simulink subsystem "tehrani_rs_calculations"  (R2020b)
settings: Solver=VariableStepAuto  StartTime=0.0  StopTime=10.0  RelTol=1e-3
values from neighbouring files (symbols this model uses):
  C_a_CO2_0 = 0.54    [model_workspace.mat]
  C_a_O2_0 = 0.1974    [model_workspace.mat]
  C_v_CO2_0 = 0.72    [model_workspace.mat]
  C_v_O2_0 = 0.13    [model_workspace.mat]
  delay_arterial = 10    [model_workspace.mat]
  delay_venous = 0    [model_workspace.mat]
settings Model: Creator=RH  LastModifiedBy=fonck

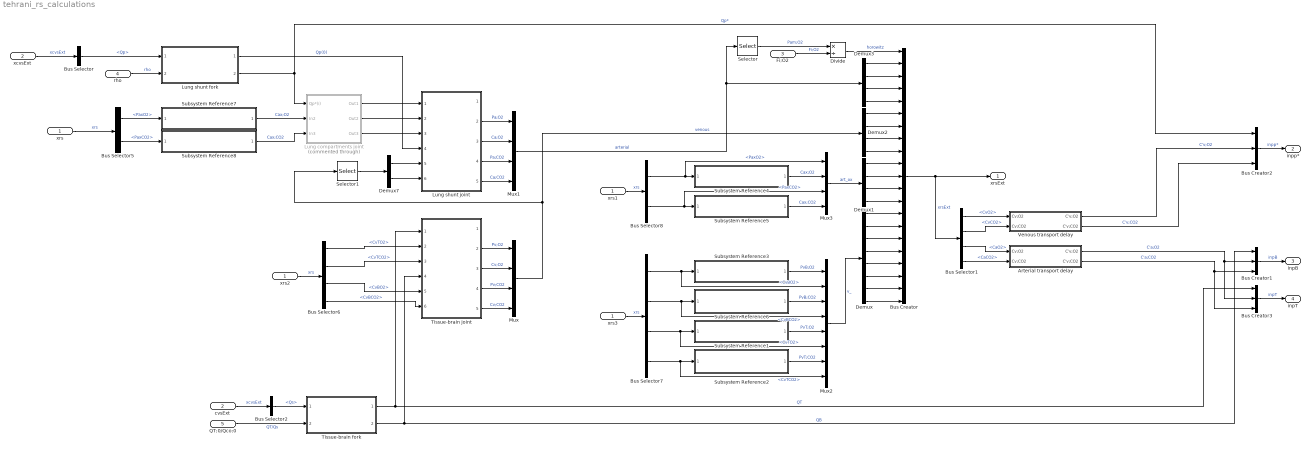
== system tehrani_rs_calculations ==
  xrs3 : Inport  OutDataTypeStr=Bus: RespiratoryState  Unit=liter/minute
  xcvsExt : Inport  Port=2  OutDataTypeStr=Bus: CardioVascularStateExtended  Unit=liter/minute
  Fi;O2 : Inport  Port=3  Unit=1
  rho : Inport  Port=4  Unit=1
  QT;0/Qco;0 : Inport  Port=5  Unit=1
  Arterial transport delay : Subsystem
  Bus Creator : BusCreator  Inputs=21  OutDataTypeStr=Bus: RespiratoryStateExtended
      settings: InheritFromInputs=off
  Bus Creator1 : BusCreator  Inputs=3  OutDataTypeStr=Bus: BloodGasFlow
      settings: InheritFromInputs=off
  Bus Creator2 : BusCreator  Inputs=3  OutDataTypeStr=Bus: BloodGasFlow
      settings: InheritFromInputs=off
  Bus Creator3 : BusCreator  Inputs=3  OutDataTypeStr=Bus: BloodGasFlow
      settings: InheritFromInputs=off
  Bus Selector : BusSelector  OutputSignals=Qp
  Bus Selector1 : BusSelector  OutputSignals=CvO2,CvCO2,CaO2,CaCO2
  Bus Selector2 : BusSelector  OutputSignals=Qs
  Bus Selector5 : BusSelector  OutputSignals=PaxO2,PaxCO2
  Bus Selector6 : BusSelector  OutputSignals=CvTO2,CvTCO2,CvBO2,CvBCO2
  Bus Selector7 : BusSelector  OutputSignals=CvBO2,CvBCO2,CvTO2,CvTCO2
  Bus Selector8 : BusSelector  OutputSignals=PaxO2,PaxCO2
  Demux : Demux  Outputs=8
  Demux1 : Demux
  Demux2 : Demux
  Demux3 : Demux
  Demux7 : Demux  Outputs=2
  Divide : Product  Inputs=*/
  Lung compartments joint : Subsystem  Commented=through
  Lung shunt fork : Subsystem  ReferencedSubsystem=blood_fork
  Lung shunt joint : Subsystem  ReferencedSubsystem=blood_joint
  Mux : Mux
  Mux1 : Mux
  Mux2 : Mux  Inputs=8
  Mux3 : Mux
  Selector : Selector  InputPortWidth=4  IndexOptions=Index vector (dialog)  Indices=[1]  OutputSizes=1
  Selector1 : Selector  InputPortWidth=4  IndexOptions=Index vector (dialog)  Indices=[2 4]  OutputSizes=1
  Subsystem Reference1 : Subsystem  ReferencedSubsystem=O2_dissociation_inv
  Subsystem Reference2 : Subsystem  ReferencedSubsystem=CO2_dissociation_inv
  Subsystem Reference3 : Subsystem  ReferencedSubsystem=O2_dissociation_inv
  Subsystem Reference4 : Subsystem  ReferencedSubsystem=O2_dissociation
  Subsystem Reference5 : Subsystem  ReferencedSubsystem=CO2_dissociation
  Subsystem Reference6 : Subsystem  ReferencedSubsystem=CO2_dissociation_inv
  Subsystem Reference7 : Subsystem  ReferencedSubsystem=O2_dissociation
  Subsystem Reference8 : Subsystem  ReferencedSubsystem=CO2_dissociation
  Tissue-brain fork : Subsystem  ReferencedSubsystem=blood_fork
  Tissue-brain joint : Subsystem  ReferencedSubsystem=blood_joint
  Venous transport delay : Subsystem
  cvsExt : InportShadow  Port=2  OutDataTypeStr=Bus: CardioVascularStateExtended  Unit=liter/minute
  xrs : InportShadow  OutDataTypeStr=Bus: RespiratoryState  Unit=liter/minute
  xrs1 : InportShadow  OutDataTypeStr=Bus: RespiratoryState  Unit=liter/minute
  xrs2 : InportShadow  OutDataTypeStr=Bus: RespiratoryState  Unit=liter/minute
  xrsExt : Outport  OutDataTypeStr=Bus: RespiratoryStateExtended
  inpp* : Outport  Port=2  OutDataTypeStr=Bus: BloodGasFlow
  inpB : Outport  Port=3  OutDataTypeStr=Bus: BloodGasFlow
  inpT : Outport  Port=4  OutDataTypeStr=Bus: BloodGasFlow
  wires:
  Arterial transport delay/1(C'v;O2) -> Bus Creator1/2, Bus Creator3/2  "C'a;O2"
  Venous transport delay/1(C'v;O2) -> Bus Creator2/2  "C'v;O2"
  Arterial transport delay/2(C'v;CO2) -> Bus Creator1/3, Bus Creator3/3  "C'a;CO2"
  Subsystem Reference3/1 -> Mux2/1  "PvB;O2"
  Subsystem Reference4/1 -> Mux3/2  "Cax;O2"
  Bus Selector1/4 -> Arterial transport delay/2(Cv;CO2)  "<CaCO2>"
  Bus Selector6/4 -> Tissue-brain joint/6  "<CvBCO2>"
  Fi;O2/1 -> Divide/2  "Fi;O2"
  Demux/7 -> Bus Creator/20
  xrs1/1 -> Bus Selector8/1  "xrs"
  Demux2/4 -> Bus Creator/9
  Demux2/2 -> Bus Creator/7
  Demux1/3 -> Bus Creator/12
  Demux1/4 -> Bus Creator/13
  Demux3/4 -> Bus Creator/5
  Demux3/1 -> Bus Creator/2
  Demux2/1 -> Bus Creator/6
  Demux2/3 -> Bus Creator/8
  Subsystem Reference1/1 -> Mux2/5  "PvT;O2"
  Demux/5 -> Bus Creator/18
  Tissue-brain joint/3 -> Mux/2  "Cv;O2"
  Bus Selector5/2 -> Subsystem Reference8/1  "<PaxCO2>"
  Subsystem Reference2/1 -> Mux2/7  "PvT;CO2"
  Demux/1 -> Bus Creator/14
  Tissue-brain joint/4 -> Mux/3  "Pv;CO2"
  Tissue-brain fork/1 -> Tissue-brain joint/1, Bus Creator3/1  "QT"
  Tissue-brain joint/5 -> Mux/4  "Cv;CO2"
  Selector1/1 -> Demux7/1
  Bus Selector7/4 -> Mux2/8, Subsystem Reference2/1  "<CvTCO2>"
  Subsystem Reference6/1 -> Mux2/3  "PvB;CO2"
  cvsExt/1 -> Bus Selector2/1  "xcvsExt"
  Demux/8 -> Bus Creator/21
  Demux/3 -> Bus Creator/16
  Demux/6 -> Bus Creator/19
  xcvsExt/1 -> Bus Selector/1  "xcvsExt"
  Lung shunt joint/3 -> Mux1/2  "Ca;O2"
  Lung shunt joint/2 -> Mux1/1  "Pa;O2"
  Demux1/1 -> Bus Creator/10
  Bus Selector8/2 -> Mux3/3, Subsystem Reference5/1  "<PaxCO2>"
  xrs3/1 -> Bus Selector7/1  "xrs"
  Lung shunt joint/4 -> Mux1/3  "Pa;CO2"
  Divide/1 -> Bus Creator/1  "horowitz"
  Bus Selector1/2 -> Venous transport delay/2(Cv;CO2)  "<CvCO2>"
  QT;0/Qco;0/1 -> Tissue-brain fork/2  "QT/Qs"
  Bus Selector1/1 -> Venous transport delay/1(Cv;O2)  "<CvO2>"
  Venous transport delay/2(C'v;CO2) -> Bus Creator2/3  "C'v;CO2"
  Mux3/1 -> Demux1/1  "art_ox"
  Tissue-brain joint/2 -> Mux/1  "Pv;O2"
  Mux2/1 -> Demux/1  "v_"
  Demux/4 -> Bus Creator/17
  Bus Selector7/2 -> Mux2/4, Subsystem Reference6/1  "<CvBCO2>"
  Demux3/2 -> Bus Creator/3
  Subsystem Reference5/1 -> Mux3/4  "Cax;CO2"
  Lung shunt fork/1 -> Lung shunt joint/4  "Qp(0)"
  Selector/1 -> Divide/1  "Pam;O2"
  Demux7/2 -> Lung shunt joint/6
  Bus Selector1/3 -> Arterial transport delay/1(Cv;O2)  "<CaO2>"
  Demux/2 -> Bus Creator/15
  Bus Selector8/1 -> Mux3/1, Subsystem Reference4/1  "<PaxO2>"
  xrs/1 -> Bus Selector5/1  "xrs"
  Bus Creator/1 -> xrsExt/1, Bus Selector1/1  "xrsExt"
  Tissue-brain fork/2 -> Bus Creator1/1, Tissue-brain joint/4  "QB"
  Bus Selector7/3 -> Mux2/6, Subsystem Reference1/1  "<CvTO2>"
  Bus Selector2/1 -> Tissue-brain fork/1  "<Qs>"
  Demux7/1 -> Lung shunt joint/5
  Bus Selector6/3 -> Tissue-brain joint/5  "<CvBO2>"
  Bus Selector6/2 -> Tissue-brain joint/3  "<CvTCO2>"
  xrs2/1 -> Bus Selector6/1  "xrs"
  rho/1 -> Lung shunt fork/2  "rho"
  Lung shunt joint/5 -> Mux1/4  "Ca;CO2"
  Bus Selector6/1 -> Tissue-brain joint/2  "<CvTO2>"
  Mux/1 -> Selector1/1, Demux2/1  "venous"
  Mux1/1 -> Selector/1, Demux3/1  "arterial"
  Bus Selector5/1 -> Subsystem Reference7/1  "<PaxO2>"
  Demux3/3 -> Bus Creator/4
  Bus Selector7/1 -> Mux2/2, Subsystem Reference3/1  "<CvBO2>"
  Demux1/2 -> Bus Creator/11
  Bus Creator2/1 -> inpp*/1  "inpp*"
  Bus Creator3/1 -> inpT/1  "inpT"
  Bus Creator1/1 -> inpB/1  "inpB"
  Bus Selector/1 -> Lung shunt fork/1  "<Qp>"
  Lung shunt fork/2 -> Bus Creator2/1, Lung compartments joint/1(Qp*(i))  "Qp*"
  Subsystem Reference7/1 -> Lung compartments joint/2(In2)  "Cax;O2"
  Subsystem Reference8/1 -> Lung compartments joint/3(In3)  "Cax;CO2"
  Lung compartments joint/1(Out1) -> Lung shunt joint/1
  Lung compartments joint/2(Out2) -> Lung shunt joint/2
  Lung compartments joint/3(Out3) -> Lung shunt joint/3

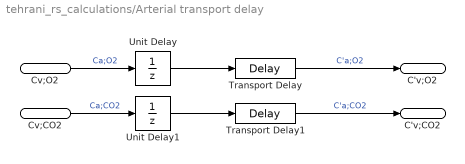
== system tehrani_rs_calculations/Arterial transport delay ==
  Cv;O2 : Inport  Unit=1
  Cv;CO2 : Inport  Port=2  Unit=1
  Transport Delay : TransportDelay  DelayTime=delay_arterial  InitialOutput=C_a_O2_0
  Transport Delay1 : TransportDelay  DelayTime=delay_arterial  InitialOutput=C_a_CO2_0
  Unit Delay : UnitDelay  InitialCondition=C_a_O2_0  SampleTime=-1  HasFrameUpgradeWarning=on
  Unit Delay1 : UnitDelay  InitialCondition=C_a_CO2_0  SampleTime=-1  HasFrameUpgradeWarning=on
  C'v;O2 : Outport  Unit=1
  C'v;CO2 : Outport  Port=2  Unit=1
  wires:
  Unit Delay1/1 -> Transport Delay1/1
  Unit Delay/1 -> Transport Delay/1
  Cv;O2/1 -> Unit Delay/1  "Ca;O2"
  Transport Delay/1 -> C'v;O2/1  "C'a;O2"
  Transport Delay1/1 -> C'v;CO2/1  "C'a;CO2"
  Cv;CO2/1 -> Unit Delay1/1  "Ca;CO2"

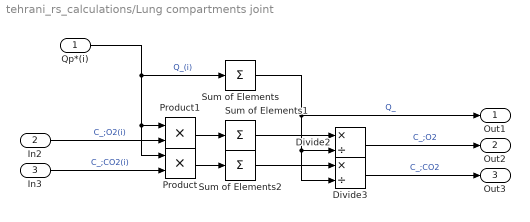
== system tehrani_rs_calculations/Lung compartments joint ==
  Qp*(i) : Inport  Unit=L/min
  In2 : Inport  Port=2  Unit=1
  In3 : Inport  Port=3  Unit=1
  Divide2 : Product  Inputs=*/
  Divide3 : Product  Inputs=*/
  Product : Product
  Product1 : Product
  Sum of Elements : Sum  Inputs=+
  Sum of Elements1 : Sum  Inputs=+
  Sum of Elements2 : Sum  Inputs=+
  Out1 : Outport  Unit=L/min
  Out2 : Outport  Port=2  Unit=1
  Out3 : Outport  Port=3  Unit=1
  wires:
  Product/1 -> Sum of Elements2/1
  Product1/1 -> Sum of Elements1/1
  In2/1 -> Product1/2  "C_;O2(i)"
  In3/1 -> Product/2  "C_;CO2(i)"
  Qp*(i)/1 -> Sum of Elements/1, Product/1, Product1/1  "Q_(i)"
  Sum of Elements2/1 -> Divide3/1
  Divide3/1 -> Out3/1  "C_;CO2"
  Divide2/1 -> Out2/1  "C_;O2"
  Sum of Elements/1 -> Divide2/2, Divide3/2, Out1/1  "Q_"
  Sum of Elements1/1 -> Divide2/1

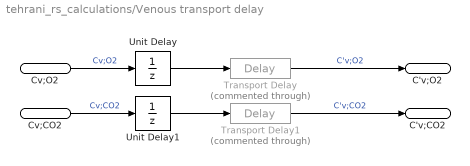
== system tehrani_rs_calculations/Venous transport delay ==
  Cv;O2 : Inport  Unit=1
  Cv;CO2 : Inport  Port=2  Unit=1
  Transport Delay : TransportDelay  Commented=through  DelayTime=delay_venous  InitialOutput=C_v_O2_0
  Transport Delay1 : TransportDelay  Commented=through  DelayTime=delay_venous  InitialOutput=C_v_CO2_0
  Unit Delay : UnitDelay  InitialCondition=C_v_O2_0  SampleTime=-1  HasFrameUpgradeWarning=on
  Unit Delay1 : UnitDelay  InitialCondition=C_v_CO2_0  SampleTime=-1  HasFrameUpgradeWarning=on
  C'v;O2 : Outport  Unit=1
  C'v;CO2 : Outport  Port=2  Unit=1
  wires:
  Unit Delay1/1 -> Transport Delay1/1
  Unit Delay/1 -> Transport Delay/1
  Cv;O2/1 -> Unit Delay/1  "Cv;O2"
  Transport Delay/1 -> C'v;O2/1  "C'v;O2"
  Transport Delay1/1 -> C'v;CO2/1  "C'v;CO2"
  Cv;CO2/1 -> Unit Delay1/1  "Cv;CO2"
